simulink model "Motor_Testing"  (R2020a)
settings: Solver=VariableStepAuto  StartTime=0.0  StopTime=10.0  RelTol=1e-3
values from neighbouring files (symbols this model uses):
  lambda_pm = 0.1194    [MotGenEvDynamicDD.sldd]
libraries: autolibdatasheetbattery x1, autolibmotorctrlr x1, autolibpmsminterior x1, simulink x1, autolibinverter x1
settings Model: Creator=Ricky  LastModifiedBy=Ricky

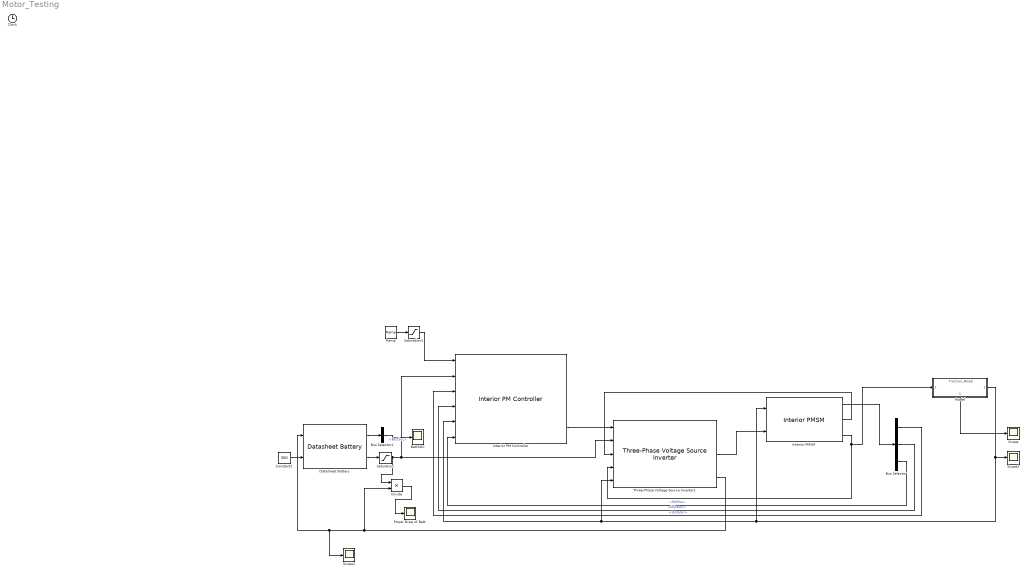
== system Motor_Testing ==
  BattSOC : Scope
  Bus Selector : BusSelector  OutputSignals=IaStator,IbStator,MtrPos
      settings: AttributesFormatString=%<OutputSignals>
  Bus Selector1 : BusSelector  OutputSignals=BattSoc
  Constant2 : Constant  Value=300
  Datasheet Battery : autolibdatasheetbattery/Datasheet Battery  CapacityCtrl=Parameter  OutputVlt=Filtered  BattChargeMax=32  Em=[2.8 3.228 3.284 3.361 3.408 3.427 3.472 3.477 3.493 3.504 3.516 3.528 3.537 3.545 3.555 3.561 3.566 3.576 3.587 3.589 3.594 3.6 3.608 3.61 3.616 3.619 3.626 3.632 3.637 3.64 3.645 3.646 3.652 3.655 3.658 3.661 3.664 3.668 3.673 3.678 3.68 3.681 3.686 3.692 3.699 3.702 3.705 3.71 3.717 3.723 3.728 3.733 3.735 3.742 3.749 3.755 3.761 3.768 3.773 3.78 3.791 3.798 3.798 3.814 3.818 3.825 3.841 3.846 3.855 3.863 3.877 3.885 3.894 3.907 3.919 3.926 3.935 3.944 3.954 3.964 3.974 3.988 3.998 4.014 4.029 4.034 4.047 4.065 4.074 4.086 4.097 4.131 4.126 4.138 4.15 4.18 4.174 4.187 4.207 4.231 4.221]  CapLUTBp=[0 0.01 0.02 0.03 0.04 0.05 0.06 0.07 0.08 0.09 0.1 0.11 0.12 0.13 0.14 0.15 0.16 0.17 0.18 0.19 0.2 0.21 0.22 0.23 0.24 0.25 0.26 0.27 0.28 0.29 0.3 0.31 0.32 0.33 0.34 0.35 0.36 0.37 0.38 0.39 0.4 0.41 0.42 0.43 0.44 0.45 0.46 0.47 0.48 0.49 0.5 0.51 0.52 0.53 0.54 0.55 0.56 0.57 0.58 0.59 0.6 0.61 0.62 0.63 0.64 0.65 0.66 0.67 0.68 0.69 0.7 0.71 0.72 0.73 0.74 0.75 0.76 0.77 0.78 0.79 0.8 0.81 0.82 0.83 0.84 0.85 0.86 0.87 0.88 0.89 0.9 0.91 0.92 0.93 0.94 0.95 0.96 0.97 0.98 0.99 1]  RInt=[0.008846 0.009319 0.009027 0.00847 0.01032 0.01314;0.006389 0.006554 0.005553 0.005525 0.006043 0.007805;0.004364 0.004101 0.00406 0.003452 0.003846 0.004517;0.002031 0.002563 0.002532 0.00246 0.002716 0.003047;0.001443 0.001825 0.001795 0.001778 0.001924 0.002234;0.0005603 0.0007192 0.0006887 0.0007557 0.0007355 0.001014;0.001028 0.001338 0.001 0.001536 0.001546 0.002789]  BattTempBp=[243.1 253.1 263.1 273.1 283.1 298.1 313.1]  CapSOCBp=[0 0.2 0.4 0.6 0.8 1]  Ns=96  Np=2  BattCapInit=26.5  Tc=1/1000  Vinit=400  RefBlkName='autolibdatasheetbattery/Datasheet Battery'
      settings: SourceProductBaseCode=PW
  Divide : Product  Inputs=**
  Interior PM Controller : autolibmotorctrlr/Interior PM Controller  control_type=Torque Control  Rs=0.02  Ld=1.7e-3  Lq=3.2e-3  lambda_pm=0.2205  PolePairs=4  Mechanical=[0.0027, 4.924e-4, 0]  T_max=120  bp=10  T_mtpa=[0 11.9390502298016 24.0093149059888 36.3310748574616 49.0066436256295 62.1183717074013 75.7302739280833 89.8912368934042 104.638389575995 119.999998392467]  id_mtpa=[-0 -0.114523352646443 -0.457989076458593 -1.030084643735447 -1.830290752214214 -2.857883673420245 -4.111938505679632 -5.591333297905697 -7.294754001684483 -9.220700201380398]  iq_mtpa=[0 18.58274403446802 37.16337191108038 55.73977348955113 74.30985061850208 92.87152301502682 111.4227340083002 129.9614561050537 148.4856963373302 166.9935013560521]  idq_limits=[-9.220699542003805 166.9935013924602 167.2478723552486]  EV_current=200  Tst=5e-5  Kp_d=2.1363  Kp_q=4.0212  Ki=25.1327  EV_motion=[20, 4, 0.8]  EV_sf=200  ba=0.40475  Ksa=10.1615  Kisa=41.2325  Ksf=1217.9727  Jcomp=0.0027  Fv=0.0004924  Fs=0  param_loss=Single efficiency measurement  eff=98  w_loss_bp=[0 200 400 600 800 1000]  T_loss_bp=[0 25 50 75 100]  losses_table=[100 100 100 100 100;100 150 200 250 300;100 200 300 400 500;100 250 400 550 700;100 300 500 700 900;100 350 600 850 1100]  w_eff_bp=[200 400 600 800 1000]  T_eff_bp=[25 50 75 100]  efficiency_table=[96.2 98.1 98.7 99;98.1 99 99.4 99.5;98.7 99.4 99.6 99.7;99 99.5 99.7 99.8;99.2 99.6 99.7 99.8]  x_w_bp=[-1000 -800 -600 -400 -200 200 400 600 800 1000]  x_T_bp=[-100 -75 -50 -25 25 50 75 100]  x_losses_mat=[200.400801603196 225.67703109328 200.803212851408 201.612903225806 199.999999999997 200 225 200;160.320641282556 180.541624874624 201.005025125625 202.020202020203 200 200 180 160;180.541624874624 180.722891566267 181.086519114686 197.568389057748 194.999999999999 179.999999999997 180 180;201.005025125625 181.086519114686 202.020202020203 193.67991845056 190 200 179.999999999997 200;202.020202020203 197.568389057748 193.67991845056 197.505197505197 190 190 194.999999999999 200;200 194.999999999999 190 190 197.505197505197 193.67991845056 197.568389057748 202.020202020203;200 179.999999999997 200 190 193.67991845056 202.020202020203 181.086519114686 201.005025125625;180 180 179.999999999997 194.999999999999 197.568389057748 181.086519114686 180.722891566267 180.541624874624;160 180 200 200 202.020202020203 201.005025125625 180.541624874624 160.320641282556;200 225 200 199.999999999997 201.612903225806 200.803212851408 225.67703109328 200.400801603196]  Tsm=5e-4
      settings: SourceProductBaseCode=PW
  Interior PMSM : autolibpmsminterior/Interior PMSM  port_config=Speed  sim_type=Continuous  Ts=0.001  P=4  Rs=.2  Ldq=[3.752e-4 4.148e-4]  KConstText=Permanent flux linkage constant (lambda_pm):  lambda_pm=0.1194  Ke=159.9771  mechanical=[0.0027, 4.924e-4, 0]  idq0=[0 0]  theta_init=0  omega_init=0  KConst=0.1194  lambda_pm_calc=0.1194  Kt=1.323  RefBlkName='autolibpmsminterior/Interior PMSM'  aMode=1
      settings: SourceProductBaseCode=PW,MT,VE,VP
  Model : ModelReference  ModelNameDialog=Traction_Model.slx  SimulationMode=Normal  ModelReferenceVersion=1.18
      settings: PortSchema="{\"entries\":[{\"content\":{\"sides\":[{\"content\":{\"connectorIds\":[\"In1\"]},\"type\":\"ConnectorPlacement.EquallySpacedRectSide\",\"uuid\":\"2c404015-eff0-4c93-ac5e-9539bc24a122\"},{\"content\":{\"connectorIds\":[\"Out2\"],\"side\":\"RIGHT\"},\"type\":\"ConnectorPlacement.EquallySpacedRectSide\",\"uuid\":\"e336d8c9-6427-42a1-9e1d-a94430f306bf\"},{\"content\":{\"connectorIds\":[],\"side\":\"TOP\"},\"type\":\"ConnectorPlacement.EquallySpacedRectSide\",\"uuid\":\"c2c69e50-9e40-41f0-95e4-225e6859d2f1\"},{\"content\":{\"connectorIds\":[\"Out1\"],\"side\":\"BOTTOM\"},\"type\":\"ConnectorPlacement.EquallySpacedRectSide\",\"uuid\":\"20194d06-13c2-41ba-a89b-c0fc39b373c7\"}]},\"type\":\"ConnectorPlacement.EquallySpacedConnector\",\"uuid\":\"37079d0d-119a-4ca4-81f9-7a10724e8df0\"}],\"packageUris\":[\"http://schema.mathworks.com/mf0/Connector/19700101\"],\"version\":\"1.0\"}"
  Power Draw of Batt : Scope
  Ramp : simulink/Sources/Ramp  slope=-50  start=0  InitialOutput=250
  Saturation : Saturate  UpperLimit=600  LowerLimit=0
  Saturation1 : Saturate  UpperLimit=250  LowerLimit=0
  Scope : Scope
  Scope1 : Scope
  Scope2 : Scope
  Three-Phase Voltage Source Inverter1 : autolibinverter/Three-Phase Voltage Source Inverter  InvrtrTmpInpEnbl=off  enable_hdl=off  model_type=Commanded phase voltage  fs=10000  w_eff_bp=[-1000 -500 0 500 1000]  n1=128  T_eff_bp=[-200 -100 0 100 200]  Temp_eff_bp=[213.15 293.15 373.15]  n2=128  ploss_table=[1 0.999 0.989 0.997 0.996;0.995 0.994 0.993 0.992 0.991;0.990 0.989 0.988 0.987 0.986;0.985 0.984 0.983 0.982 0.981;0.980 0.979 0.978 0.977 0.976]  ploss_table_3d=cat(3,0.95*[1 0.999 0.989 0.997 0.996;0.995 0.994 0.993 0.992 0.991;0.990 0.989 0.988 0.987 0.986;0.985 0.984 0.983 0.982 0.981;0.980 0.979 0.978 0.977 0.976],[1 0.999 0.989 0.997 0.996;0.995 0.994 0.993 0.992 0.991;0.990 0.989 0.988 0.987 0.986;0.985 0.984 0.983 0.982 0.981;0.980 0.979 0.978 0.977 0.976],0.92*[1 0.999 0.989 0.997 0.996;0.995 0.994 0.993 0.992 0.991;0.990 0.989 0.988 0.987 0.986;0.985 0.984 0.983 0.982 0.981;0.980 0.979 0.978 0.977 0.976])  preExtrapFlag=off  u1max=1000  u1min=-1000  u2max=200  u2min=-200  intPrec=23  RefBlkName='autolibmappedmotor/Mapped Motor'  CalLossMapData={}  CalLossWithTempMapData={}
      settings: SourceProductBaseCode=PW,MT,VE,VP
  Clock : Clock
      settings: IOType=siggen
  wires:
  Ramp/1 -> Saturation1/1
  Interior PM Controller/3 -> Three-Phase Voltage Source Inverter1/1
  Three-Phase Voltage Source Inverter1/2 -> Interior PMSM/2
  Interior PMSM/3 -> Model/1, Three-Phase Voltage Source Inverter1/4
  Interior PMSM/2 -> Three-Phase Voltage Source Inverter1/3
  Interior PMSM/1 -> Bus Selector/1
  Bus Selector/1 -> Interior PM Controller/3  "<IaStator>"
  Bus Selector/2 -> Interior PM Controller/4  "<IbStator>"
  Bus Selector/3 -> Interior PM Controller/6  "<MtrPos>"
  Model/1 -> Scope/1
  Constant2/1 -> Datasheet Battery/2
  Datasheet Battery/2 -> Saturation/1
  Three-Phase Voltage Source Inverter1/3 -> Divide/2, Scope1/1, Datasheet Battery/1
  Datasheet Battery/1 -> Bus Selector1/1
  Bus Selector1/1 -> BattSOC/1  "<BattSoc>"
  Saturation/1 -> Divide/1, Three-Phase Voltage Source Inverter1/2, Interior PM Controller/2
  Model/2 -> Scope2/1, Interior PMSM/1, Three-Phase Voltage Source Inverter1/5, Interior PM Controller/5
  Saturation1/1 -> Interior PM Controller/1
  Divide/1 -> Power Draw of Batt/1
